simulink model "PMSM_FOC_Algorithm"  (R2024b)
settings: Solver=FixedStepAuto  StartTime=0.0  StopTime=1  FixedStep=1e-6  RelTol=1e-3
model workspace (MAT data in the model file):
  B = 0
  Current_Filter_On = 1
  F = 10000
  J = 5.8e-05
  Ls = 0.0005125
  Pn = 5
  Rs = 0.1445
  T_deadband = 3e-06
  Ts = 5e-05
  Vdc = 48
  id_ki = 0.01
  id_kp = 0.8
  iq_ki = 0.01
  iq_kp = 1.2
  psi_f = 0.0113
libraries: simulink x2, slpidlib x2, spsDCVoltageSourceLib x1, spsOnDelayLib x1, spsPermanentMagnetSynchronousMachineLib x1, spsTwoLevelConverterLib x1, spspowerguiLib x1
settings Model: Creator=A  LastModifiedBy=31904
settings OptimizationCC: ReuseModelBlockBuffer=off
settings ModelReferenceCC: EnableRefExpFcnMdlSchedulingChecks=on
settings RTWCC: GPUComputeCapability=3.5

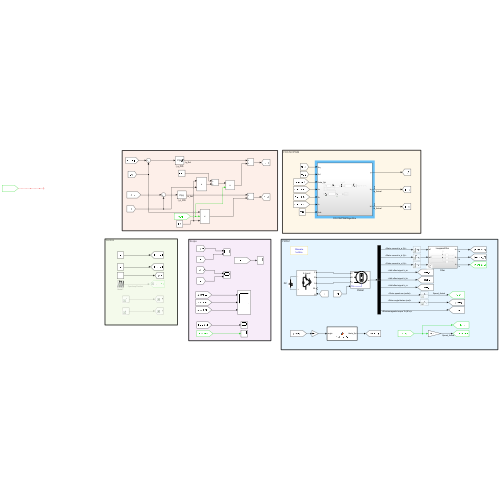
[thumbnail: Simulink's stored preview of the top-level diagram]
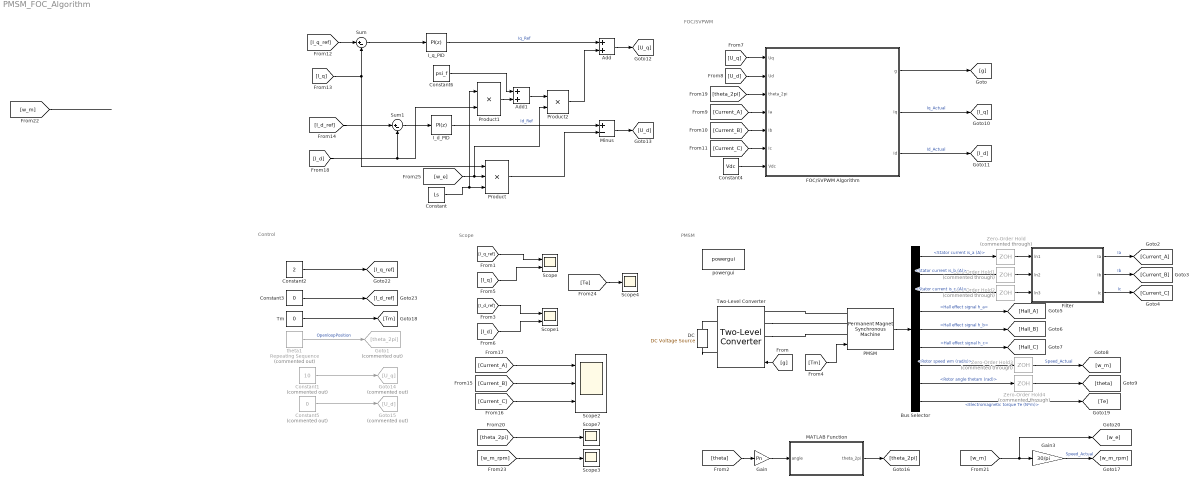
== system PMSM_FOC_Algorithm ==
  note: Scope
  note: Control
  note: FOC/SVPWM
  note: PMSM
  Add : Sum
  Add1 : Sum
  Bus Selector : BusSelector  OutputSignals=Stator current is_a (A),Stator current is_b (A),Stator current is_c (A),Hall effect signal h_a,Hall effect signal h_b,Hall effect signal h_c,Rotor speed wm (rad/s),Rotor angle thetam (rad),Electromagnetic torque Te (N*m)
  Constant : Constant  Value=Ls
  Constant1 : Constant  Commented=on  Value=10
  Constant2 : Constant  Value=2
  Constant3 : Constant  Value=0
  Constant4 : Constant  Value=Vdc
  Constant5 : Constant  Commented=on  Value=0
  Constant6 : Constant  Value=psi_f
  DC : spsDCVoltageSourceLib/DC Voltage Source  Amplitude=Vdc  Measurements=None
  FOC/SVPWM Algorithm : Subsystem
  Filter : Subsystem  Variant=on
  Gain : Gain  Gain=Pn
  Gain3 : Gain  Gain=30/pi
  Goto1 : Goto  Commented=on  GotoTag=theta_2pi
  Goto14 : Goto  Commented=on  GotoTag=U_q
  Goto15 : Goto  Commented=on  GotoTag=U_d
  I_d_PID : slpidlib/PID Controller  Controller=PI  Form=Parallel  TimeDomain=Discrete-time  UseExternalTs=off  SampleTime=-1  IntegratorMethod=Forward Euler  FilterMethod=Forward Euler  ControllerParametersSource=internal  P=id_kp  I=id_ki  UseKiTs=off  D=0  UseExternalDerivativeSource=off  N=100  UseFilter=on  TunerSelectOption=Transfer Function Based (PID Tuner App)  InitialConditionSource=internal  InitialConditionForIntegrator=0  InitialConditionForFilter=0  DifferentiatorICPrevScaledInput=0  ExternalReset=none  TrackingMode=off  Kt=1  LimitOutput=off  SatLimitsSource=internal  UpperSaturationLimit=10  LowerSaturationLimit=0  LinearizeAsGain=on  AntiWindupMode=none  Kb=1  LimitIntegrator=off  UpperIntegratorSaturationLimit=inf  LowerIntegratorSaturationLimit=-inf  POutMin=[]  POutMax=[]  IOutMin=[]  IOutMax=[]  DOutMin=[]  DOutMax=[]  NOutMin=[]  NOutMax=[]  SumOutMin=[]  SumOutMax=[]  SaturationOutMin=[]  SaturationOutMax=[]  PParamMin=[]  PParamMax=[]  IParamMin=[]  IParamMax=[]  DParamMin=[]  DParamMax=[]  NParamMin=[]  NParamMax=[]  KbParamMin=[]  KbParamMax=[]  KtParamMin=[]  KtParamMax=[]  KbOutMin=[]  KbOutMax=[]  KtOutMin=[]  KtOutMax=[]  IntegratorOutMin=[]  IntegratorOutMax=[]  FilterOutMin=[]  FilterOutMax=[]  SumI1OutMin=[]  SumI1OutMax=[]  SumI2OutMin=[]  SumI2OutMax=[]  SumI3OutMin=[]  SumI3OutMax=[]  SumI4OutMin=[]  SumI4OutMax=[]  SumDOutMin=[]  SumDOutMax=[]  DifferentiatorOutMin=[]  DifferentiatorOutMax=[]  FilterDiffOutCoefMin=[]  FilterDiffOutCoefMax=[]  ReciprocalOutMin=[]  ReciprocalOutMax=[]  SumDenOutMin=[]  SumDenOutMax=[]  SumNumOutMin=[]  SumNumOutMax=[]  DivideOutMin=[]  DivideOutMax=[]  UdiffTsProdOutMin=[]  UdiffTsProdOutMax=[]  NTsProdOutMin=[]  NTsProdOutMax=[]  UintegralTsProdOutMin=[]  UintegralTsProdOutMax=[]  UngainTsProdOutMin=[]  UngainTsProdOutMax=[]  ClampingZeroOutDataTypeStr=Inherit: Inherit via back propagation  ClampingZeroOutMin=[]  ClampingZeroOutMax=[]  FilterDenConstantOutDataTypeStr=Inherit: Inherit via back propagation  FilterDenConstantOutMin=[]  FilterDenConstantOutMax=[]  PCopyOutDataTypeStr=Inherit: Inherit via back propagation  PCopyOutMin=[]  PCopyOutMax=[]  NCopyOutDataTypeStr=Inherit: Inherit via back propagation  NCopyOutMin=[]  NCopyOutMax=[]  IntegratorContinuousStateAttributes=''  IntegratorStateMustResolveToSignalObject=off  IntegratorRTWStateStorageClass=Auto  FilterContinuousStateAttributes=''  FilterStateMustResolveToSignalObject=off  FilterRTWStateStorageClass=Auto  ParallelPVariant=InternalParameters  IdealPVariant=Disabled  IVariant=InternalParameters  DVariant=Disabled  IntegratorVariant=Discrete  SatVariant=Disabled  AWVariant=Passthrough  PCopyVariant=Disabled  TRVariant=Disabled  FdbkBlocksVariant=Forward  IdealPFdbkVariant=Disabled  SatFdbkVariant=Disabled  DerivativeFilterVariant=Disabled  NVariant=Disabled  NCopyVariant=Disabled_SignalSpec  FilterICVariant=Disabled  IntegratorICVariant=InternalICs  ExternalResetVariant=Disabled  TRSumVariant=Passthrough  SumFdbkVariant=Disabled  SumVariant=Sum_PI  TsampFilterVariant=InternalTs  TsampNgainVariant=Passthrough  TsampIntegralVariant=Disabled_SignalSpec  ExternalSaturationOutDataTypeStr=Inherit: Same as second input  DerivativeSourceVariant=Disabled  PreIntVariant=InternalPreInt
  I_q_PID : slpidlib/PID Controller  Controller=PI  Form=Parallel  TimeDomain=Discrete-time  UseExternalTs=off  SampleTime=-1  IntegratorMethod=Forward Euler  FilterMethod=Forward Euler  ControllerParametersSource=internal  P=iq_kp  I=iq_ki  UseKiTs=off  D=0  UseExternalDerivativeSource=off  N=100  UseFilter=on  TunerSelectOption=Transfer Function Based (PID Tuner App)  InitialConditionSource=internal  InitialConditionForIntegrator=0  InitialConditionForFilter=0  DifferentiatorICPrevScaledInput=0  ExternalReset=none  TrackingMode=off  Kt=1  LimitOutput=on  SatLimitsSource=internal  UpperSaturationLimit=Vdc  LowerSaturationLimit=0  LinearizeAsGain=on  AntiWindupMode=back-calculation  Kb=1  LimitIntegrator=off  UpperIntegratorSaturationLimit=inf  LowerIntegratorSaturationLimit=-inf  POutMin=[]  POutMax=[]  IOutMin=[]  IOutMax=[]  DOutMin=[]  DOutMax=[]  NOutMin=[]  NOutMax=[]  SumOutMin=[]  SumOutMax=[]  SaturationOutMin=[]  SaturationOutMax=[]  PParamMin=[]  PParamMax=[]  IParamMin=[]  IParamMax=[]  DParamMin=[]  DParamMax=[]  NParamMin=[]  NParamMax=[]  KbParamMin=[]  KbParamMax=[]  KtParamMin=[]  KtParamMax=[]  KbOutMin=[]  KbOutMax=[]  KtOutMin=[]  KtOutMax=[]  IntegratorOutMin=[]  IntegratorOutMax=[]  FilterOutMin=[]  FilterOutMax=[]  SumI1OutMin=[]  SumI1OutMax=[]  SumI2OutMin=[]  SumI2OutMax=[]  SumI3OutMin=[]  SumI3OutMax=[]  SumI4OutMin=[]  SumI4OutMax=[]  SumDOutMin=[]  SumDOutMax=[]  DifferentiatorOutMin=[]  DifferentiatorOutMax=[]  FilterDiffOutCoefMin=[]  FilterDiffOutCoefMax=[]  ReciprocalOutMin=[]  ReciprocalOutMax=[]  SumDenOutMin=[]  SumDenOutMax=[]  SumNumOutMin=[]  SumNumOutMax=[]  DivideOutMin=[]  DivideOutMax=[]  UdiffTsProdOutMin=[]  UdiffTsProdOutMax=[]  NTsProdOutMin=[]  NTsProdOutMax=[]  UintegralTsProdOutMin=[]  UintegralTsProdOutMax=[]  UngainTsProdOutMin=[]  UngainTsProdOutMax=[]  ClampingZeroOutDataTypeStr=Inherit: Inherit via back propagation  ClampingZeroOutMin=[]  ClampingZeroOutMax=[]  FilterDenConstantOutDataTypeStr=Inherit: Inherit via back propagation  FilterDenConstantOutMin=[]  FilterDenConstantOutMax=[]  PCopyOutDataTypeStr=Inherit: Inherit via back propagation  PCopyOutMin=[]  PCopyOutMax=[]  NCopyOutDataTypeStr=Inherit: Inherit via back propagation  NCopyOutMin=[]  NCopyOutMax=[]  IntegratorContinuousStateAttributes=''  IntegratorStateMustResolveToSignalObject=off  IntegratorRTWStateStorageClass=Auto  FilterContinuousStateAttributes=''  FilterStateMustResolveToSignalObject=off  FilterRTWStateStorageClass=Auto  ParallelPVariant=InternalParameters  IdealPVariant=Disabled  IVariant=InternalParameters  DVariant=Disabled  IntegratorVariant=Discrete  SatVariant=Enabled  AWVariant=BackCalculation  PCopyVariant=Disabled  TRVariant=Disabled  FdbkBlocksVariant=Forward  IdealPFdbkVariant=Disabled  SatFdbkVariant=Disabled  DerivativeFilterVariant=Disabled  NVariant=Disabled  NCopyVariant=Disabled_SignalSpec  FilterICVariant=Disabled  IntegratorICVariant=InternalICs  ExternalResetVariant=Disabled  TRSumVariant=Passthrough  SumFdbkVariant=Disabled  SumVariant=Sum_PI  TsampFilterVariant=InternalTs  TsampNgainVariant=Passthrough  TsampIntegralVariant=Disabled_SignalSpec  ExternalSaturationOutDataTypeStr=Inherit: Same as second input  DerivativeSourceVariant=Disabled  PreIntVariant=InternalPreInt
  MATLAB Function : MATLAB Function  TreatAsAtomicUnit=on
  Minus : Sum  Inputs=+-
  PMSM : spsPermanentMagnetSynchronousMachineLib/Permanent Magnet Synchronous Machine  NbPhases=3  FluxDistribution=Sinusoidal  RotorType=Round  MechanicalLoad=Torque Tm  PresetModel=No  ShowDetailedParameters=on  MeasurementBus=off  Resistance=Rs  Inductance=8.5e-3  dqInductances=[8.5e-3,8.5e-3]  La=Ls  MachineConstant=Flux linkage established by magnets (V.s)  Flux=psi_f  VoltageCst=10.248  TorqueCst=0.08475  Flat=120  Mechanical=[J B Pn 0]  PolePairs=4  InitialConditions=[0,0, 0,0]  InitialConditions5ph=[0 0 0 0 0 0]  RefAngle=Aligned with phase A axis (original Park)  IterativeDiscreteModel=Trapezoidal non iterative  TsBlock=-1  TsPowergui=0
  Product : Product  Inputs=3
  Product1 : Product
  Product2 : Product
  Scope : Scope  NumInputPorts=2
  Scope1 : Scope  NumInputPorts=2
  Scope2 : Scope  NumInputPorts=3
  Scope3 : Scope
  Scope4 : Scope
  Scope7 : Scope
  Sum : Sum  Inputs=|+-
  Sum1 : Sum  Inputs=|+-
  Tm : Constant  Value=0
  Two-Level Converter : spsTwoLevelConverterLib/Two-Level Converter  ModelType=Switching devices  Ron=1e-3  Rs=1e6  Cs=inf  Vforward=[0,0]  Ron_Diode=1e-3  Rs_Diode=1e6  Cs_Diode=inf  Vf_Diode=1e-3  Rs_CurrentSource=inf  Ron_ACsource=1e-3
  Zero-Order Hold{,1..4} (5 alike) : ZeroOrderHold  Commented=through  SampleTime=1/F
  powergui : spspowerguiLib/powergui  Priority=1  SimulationMode=Discrete  SampleTime=1e-6  frequency=60  Iterations=50  frequencyindice=0  Pbase=100e6  ErrMax=1e-4  UnitsV=kV  UnitsW=MW  buscounter=0  FunctionMessages=off  echomessages=off  EnableUseOfTLC=off  CurrentSourceSwitches=off  DisableSnubberDevices=off  DisableRonSwitches=off  DisableVfSwitches=off  DisplayEquations=off  AutomaticDiscreteSolvers=off  SolverType=Tustin/Backward Euler (TBE)  Interpol=off  ExternalGateDelay=off  methode=off  Ts=100  x0status=blocks  SPID=on  SwTol=0  HookPort=off  NonlinearTolerance=1e-4  nMaxIteration=100  ContinueOnMaxIteration=off  RestoreLinks=warning  ResistiveCurrentMeasurement=off  Frange=[0:2:500]  Ylog=off  Xlog=on  ShowGrid=off  save=off  variable=ZData  structure=0  ZoomFFT=off  StartTime=0.0  cycles=1  DisplayStyle=1  fundamental=60  FreqAxis=off  MaxFrequency=1000  frequencyindicesteady=1  RmsSteady=1  display=off
  theta1 : simulink/Sources/Repeating Sequence  Commented=on  rep_seq_t=[0 0.1]  rep_seq_y=[0 2*pi]
  wires:
  Constant4/1 -> FOC/SVPWM Algorithm/7(Vdc)
  [theta_2pi] -> FOC/SVPWM Algorithm/3(theta_2pi)
  FOC/SVPWM Algorithm/3(Id) -> [I_d]  "Id_Actual"
  [U_d] -> FOC/SVPWM Algorithm/2(Ud)
  [U_q] -> FOC/SVPWM Algorithm/1(Uq)
  [Current_A] -> FOC/SVPWM Algorithm/4(Ia)
  [Current_C] -> FOC/SVPWM Algorithm/6(Ic)
  FOC/SVPWM Algorithm/2(Iq) -> [I_q]  "Iq_Actual"
  [Current_B] -> FOC/SVPWM Algorithm/5(Ib)
  Zero-Order Hold4/1 -> [theta]
  Bus Selector/1 -> Zero-Order Hold/1  "<Stator current is_a (A)>"
  Zero-Order Hold/1 -> Filter/1(ln1)
  Zero-Order Hold1/1 -> Filter/2(ln2)
  Bus Selector/4 -> [Hall_A]  "<Hall effect signal h_a>"
  [theta] -> Gain/1
  Bus Selector/2 -> Zero-Order Hold1/1  "<Stator current is_b (A)>"
  [g] -> Two-Level Converter/1
  Bus Selector/3 -> Zero-Order Hold2/1  "<Stator current is_c (A)>"
  [Tm] -> PMSM/1
  Zero-Order Hold3/1 -> [w_m]  "Speed_Actual"
  Bus Selector/8 -> Zero-Order Hold4/1  "<Rotor angle thetam (rad)>"
  MATLAB Function/1(theta_2pi) -> [theta_2pi]
  Bus Selector/7 -> Zero-Order Hold3/1  "<Rotor speed wm (rad/s)>"
  PMSM/1 -> Bus Selector/1
  Bus Selector/5 -> [Hall_B]  "<Hall effect signal h_b>"
  Zero-Order Hold2/1 -> Filter/3(ln3)
  Bus Selector/6 -> [Hall_C]  "<Hall effect signal h_c>"
  Constant3/1 -> [I_d_ref]
  Constant2/1 -> [I_q_ref]
  [I_q_ref] -> Scope/1
  [I_q] -> Scope/2
  [I_d_ref] -> Scope1/1
  [I_d] -> Scope1/2
  I_q_PID/1 -> Add/1  "Iq_Ref"
  [I_q_ref] -> Sum/1
  [I_q] -> Sum/2, Product/1
  Sum/1 -> I_q_PID/1
  [Current_C] -> Scope2/3
  [Current_B] -> Scope2/2
  [Current_A] -> Scope2/1
  [theta_2pi] -> Scope7/1
  Filter/1(Ia) -> [Current_A]  "Ia"
  Filter/2(Ib) -> [Current_B]  "Ib"
  Filter/3(Ic) -> [Current_C]  "Ic"
  FOC/SVPWM Algorithm/1(g) -> [g]
  theta1/1 -> Goto1/1  "OpenloopPosition"
  Sum1/1 -> I_d_PID/1
  I_d_PID/1 -> Minus/1  "Id_Ref"
  [I_d] -> Product1/2, Sum1/2
  [I_d_ref] -> Sum1/1
  Constant5/1 -> Goto15/1
  Constant1/1 -> Goto14/1
  [w_m] -> [w_e], Gain3/1
  Gain3/1 -> [w_m_rpm]  "Speed_Actual"
  [w_m] -> ?
  [w_m_rpm] -> Scope3/1
  Gain/1 -> MATLAB Function/1(angle)
  Tm/1 -> [Tm]
  Bus Selector/9 -> [Te]  "<Electromagnetic torque Te (N*m)>"
  [Te] -> Scope4/1
  [w_e] -> Product2/2, Product/2
  Constant/1 -> Product1/1, Product/3
  Product/1 -> Minus/2
  Minus/1 -> [U_d]
  Product1/1 -> Add1/2
  Constant6/1 -> Add1/1
  Add1/1 -> Product2/1
  Product2/1 -> Add/2
  Add/1 -> [U_q]
  connections:
  DC/LConn1 -- Two-Level Converter/RConn2
  DC/RConn1 -- Two-Level Converter/RConn1
  PMSM/LConn3 -- Two-Level Converter/LConn3
  Two-Level Converter/LConn1 -- PMSM/LConn1
  Two-Level Converter/LConn2 -- PMSM/LConn2

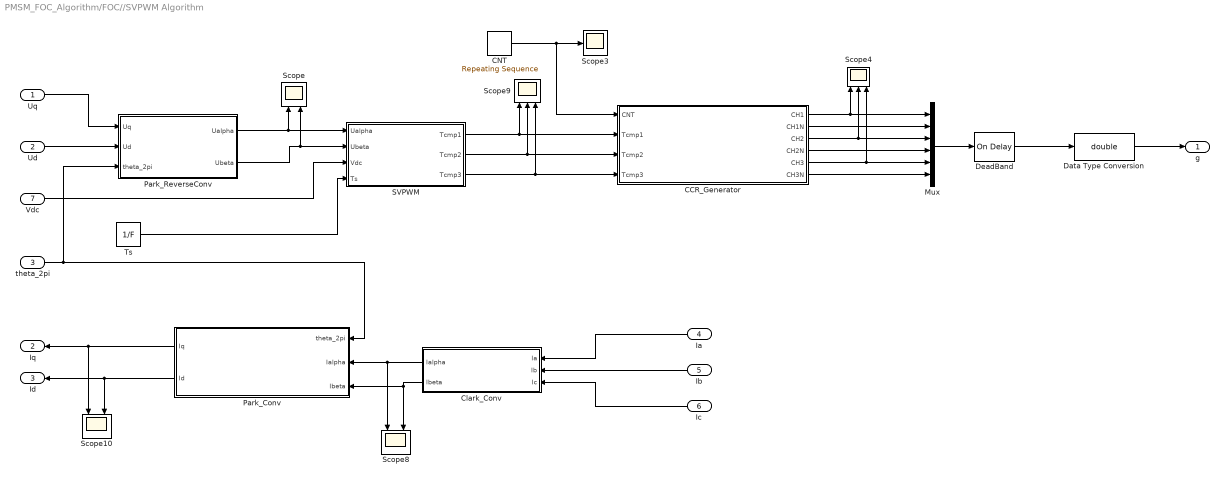
== system PMSM_FOC_Algorithm/FOC//SVPWM Algorithm ==
  Uq : Inport
  Ud : Inport  Port=2
  theta_2pi : Inport  Port=3
  Ia : Inport  Port=4
  Ib : Inport  Port=5
  Ic : Inport  Port=6
  Vdc : Inport  Port=7
  CCR_Generator : MATLAB Function  TreatAsAtomicUnit=on
  CNT : simulink/Sources/Repeating Sequence  rep_seq_t=[0 1/(2*F) 1/F]  rep_seq_y=[0 1/(2*F) 0]
  Clark_Conv : Subsystem
  Data Type Conversion : DataTypeConversion  OutDataTypeStr=double  SaturateOnIntegerOverflow=off  RndMeth=Floor
  DeadBand : spsOnDelayLib/On Delay  DelayType=On delay  delay=T_deadband  ic=0  Ts=0
  Mux : Mux  Inputs=6
  Park_Conv : Subsystem
  Park_ReverseConv : Subsystem
  SVPWM : Subsystem
  Scope : Scope  NumInputPorts=2
  Scope10 : Scope  NumInputPorts=2
  Scope3 : Scope
  Scope4 : Scope  NumInputPorts=3
  Scope8 : Scope  NumInputPorts=2
  Scope9 : Scope  NumInputPorts=3
  Ts : Constant  Value=1/F
  g : Outport
  Iq : Outport  Port=2
  Id : Outport  Port=3
  wires:
  Uq/1 -> Park_ReverseConv/1(Uq)
  SVPWM/3(Tcmp3) -> CCR_Generator/4(Tcmp3), Scope9/3
  Clark_Conv/1(Ialpha) -> Park_Conv/2(Ialpha), Scope8/1
  CCR_Generator/3(CH2) -> Mux/3, Scope4/2
  SVPWM/2(Tcmp2) -> CCR_Generator/3(Tcmp2), Scope9/2
  CCR_Generator/2(CH1N) -> Mux/2
  theta_2pi/1 -> Park_Conv/1(theta_2pi), Park_ReverseConv/3(theta_2pi)
  CCR_Generator/5(CH3) -> Mux/5, Scope4/3
  SVPWM/1(Tcmp1) -> CCR_Generator/2(Tcmp1), Scope9/1
  Clark_Conv/2(Ibeta) -> Park_Conv/3(Ibeta), Scope8/2
  CCR_Generator/4(CH2N) -> Mux/4
  Park_ReverseConv/1(Ualpha) -> SVPWM/1(Ualpha), Scope/1
  CCR_Generator/6(CH3N) -> Mux/6
  Mux/1 -> DeadBand/1
  Park_ReverseConv/2(Ubeta) -> Scope/2, SVPWM/2(Ubeta)
  CNT/1 -> Scope3/1, CCR_Generator/1(CNT)
  Park_Conv/2(Id) -> Scope10/2, Id/1
  CCR_Generator/1(CH1) -> Mux/1, Scope4/1
  Ud/1 -> Park_ReverseConv/2(Ud)
  Park_Conv/1(Iq) -> Scope10/1, Iq/1
  Data Type Conversion/1 -> g/1
  Vdc/1 -> SVPWM/3(Vdc)
  Ic/1 -> Clark_Conv/3(Ic)
  Ib/1 -> Clark_Conv/2(Ib)
  Ia/1 -> Clark_Conv/1(Ia)
  Ts/1 -> SVPWM/4(Ts)
  DeadBand/1 -> Data Type Conversion/1

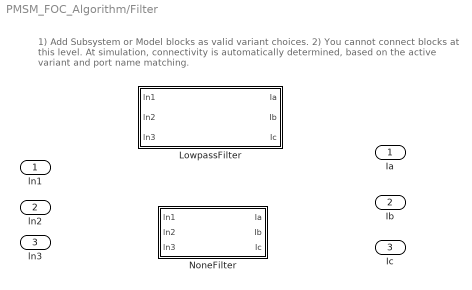
== system PMSM_FOC_Algorithm/Filter ==
  note: 1) Add Subsystem or Model blocks as valid variant choices.
      | 2) You cannot connect blocks at this level. At simulation, connectivity is automatically
      | determined, based on the active variant and port name matching.
  ln1 : Inport
  ln2 : Inport  Port=2
  ln3 : Inport  Port=3
  LowpassFilter : Subsystem  VariantControl=Current_Filter_On==1
  NoneFilter : Subsystem  VariantControl=Current_Filter_On==0
  Ia : Outport
  Ib : Outport  Port=2
  Ic : Outport  Port=3

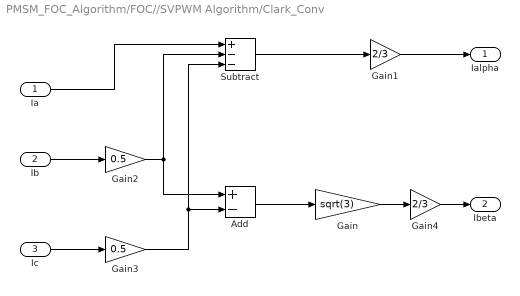
== system PMSM_FOC_Algorithm/FOC//SVPWM Algorithm/Clark_Conv ==
  Ia : Inport
  Ib : Inport  Port=2
  Ic : Inport  Port=3
  Add : Sum  Inputs=+-  OutDataTypeStr=double
  Gain : Gain  Gain=sqrt(3)  ParamDataTypeStr=double
  Gain1 : Gain  Gain=2/3
  Gain2 : Gain  Gain=0.5
  Gain3 : Gain  Gain=0.5
  Gain4 : Gain  Gain=2/3
  Subtract : Sum  Inputs=+--  OutDataTypeStr=double
  Ialpha : Outport
  Ibeta : Outport  Port=2
  wires:
  Ia/1 -> Subtract/1
  Ib/1 -> Gain2/1
  Add/1 -> Gain/1
  Gain/1 -> Gain4/1
  Ic/1 -> Gain3/1
  Gain2/1 -> Subtract/2, Add/1
  Gain3/1 -> Subtract/3, Add/2
  Subtract/1 -> Gain1/1
  Gain1/1 -> Ialpha/1
  Gain4/1 -> Ibeta/1

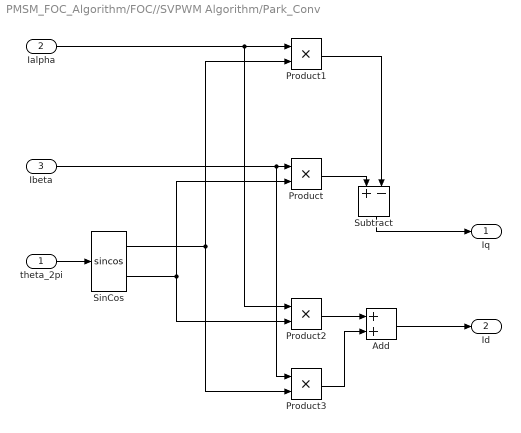
== system PMSM_FOC_Algorithm/FOC//SVPWM Algorithm/Park_Conv ==
  theta_2pi : Inport
  Ialpha : Inport  Port=2
  Ibeta : Inport  Port=3
  Add : Sum
  Product{,1..3} (4 alike) : Product
  SinCos : Trigonometry  Operator=sincos
  Subtract : Sum  Inputs=+-
  Iq : Outport
  Id : Outport  Port=2
  wires:
  Ialpha/1 -> Product1/1, Product2/1
  Ibeta/1 -> Product3/1, Product/1
  theta_2pi/1 -> SinCos/1
  SinCos/2 -> Product2/2, Product/2
  SinCos/1 -> Product3/2, Product1/2
  Product1/1 -> Subtract/2
  Subtract/1 -> Iq/1
  Product/1 -> Subtract/1
  Product2/1 -> Add/1
  Product3/1 -> Add/2
  Add/1 -> Id/1

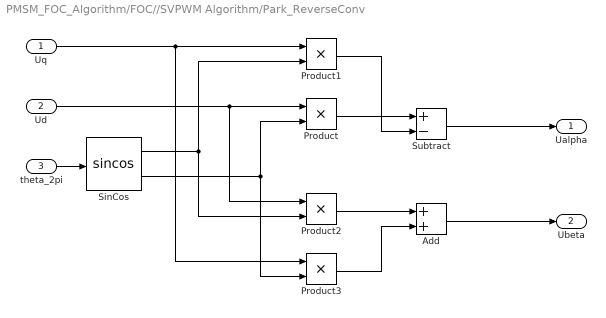
== system PMSM_FOC_Algorithm/FOC//SVPWM Algorithm/Park_ReverseConv ==
  Uq : Inport
  Ud : Inport  Port=2
  theta_2pi : Inport  Port=3
  Add : Sum
  Product{,1..3} (4 alike) : Product
  SinCos : Trigonometry  Operator=sincos
  Subtract : Sum  Inputs=+-
  Ualpha : Outport
  Ubeta : Outport  Port=2
  wires:
  Uq/1 -> Product3/1, Product1/1
  Ud/1 -> Product2/1, Product/1
  SinCos/2 -> Product3/2, Product/2
  Product/1 -> Subtract/1
  SinCos/1 -> Product2/2, Product1/2
  Product1/1 -> Subtract/2
  Subtract/1 -> Ualpha/1
  Product2/1 -> Add/1
  Product3/1 -> Add/2
  Add/1 -> Ubeta/1
  theta_2pi/1 -> SinCos/1

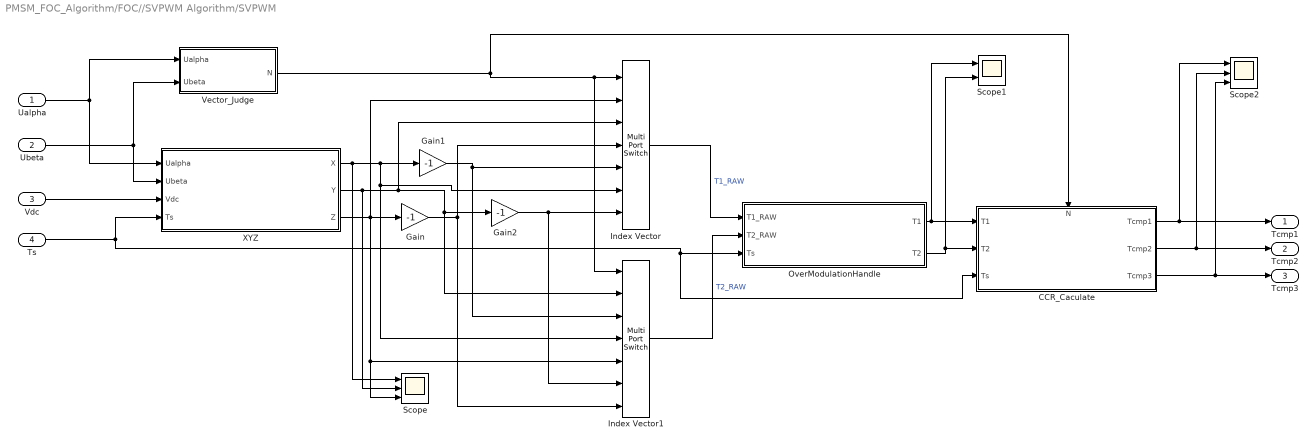
== system PMSM_FOC_Algorithm/FOC//SVPWM Algorithm/SVPWM ==
  Ualpha : Inport
  Ubeta : Inport  Port=2
  Vdc : Inport  Port=3
  Ts : Inport  Port=4
  CCR_Caculate : Subsystem
      settings: PortSchema="{\"entries\":[{\"content\":{\"sides\":[{\"content\":{\"connectorIds\":[\"In1\",\"In2\",\"In3\"]},\"type\":\"ConnectorPlacement.EquallySpacedRectSide\",\"uuid\":\"41d89106-695f-4d7e-9c99-c52170b99868\"},{\"content\":{\"connectorIds\":[\"Out1\",\"Out2\",\"Out3\"],\"side\":\"RIGHT\"},\"type\":\"ConnectorPlacement.EquallySpacedRectSide\",\"uuid\":\"0fa1e6b9-7088-4c16-9dd3-c016449aae3e\"},{\"content\":{\"connectorIds\":[\"In4\"],\"side\":\"TOP\"},\"type\":\"ConnectorPlacement.EquallySpacedRectSide\",\"uuid\":\"6b702c00-29ab-49c7-a344-eb6fce3368af\"}]},\"type\":\"ConnectorPlacement.EquallySpacedConnector\",\"uuid\":\"c2f99839-550c-47c5-98fa-a115626cfb71\"}],\"packageUris\":[\"http://schema.mathworks.com/mf0/Connector/R2020b\"],\"version\":\"1.0\"}"
  Gain : Gain  Gain=-1
  Gain1 : Gain  Gain=-1
  Gain2 : Gain  Gain=-1
  Index Vector : MultiPortSwitch  Inputs=6  SaturateOnIntegerOverflow=off  InputSameDT=off
  Index Vector1 : MultiPortSwitch  Inputs=6  SaturateOnIntegerOverflow=off  InputSameDT=off
  OverModulationHandle : MATLAB Function  TreatAsAtomicUnit=on
  Scope : Scope  NumInputPorts=3
  Scope1 : Scope  NumInputPorts=2
  Scope2 : Scope  NumInputPorts=3
  Vector_Judge : Subsystem
  XYZ : Subsystem
  Tcmp1 : Outport
  Tcmp2 : Outport  Port=2
  Tcmp3 : Outport  Port=3
  wires:
  Ualpha/1 -> Vector_Judge/1(Ualpha), XYZ/1(Ualpha)
  Ubeta/1 -> Vector_Judge/2(Ubeta), XYZ/2(Ubeta)
  Vdc/1 -> XYZ/3(Vdc)
  Ts/1 -> CCR_Caculate/3(Ts), OverModulationHandle/3(Ts), XYZ/4(Ts)
  Vector_Judge/1(N) -> Index Vector1/1, Index Vector/1, CCR_Caculate/4(N)
  Index Vector1/1 -> OverModulationHandle/2(T2_RAW)  "T2_RAW"
  XYZ/3(Z) -> Scope/3, Index Vector1/5, Index Vector/2, Gain/1
  XYZ/2(Y) -> Scope/2, Index Vector1/2, Gain2/1, Index Vector/3
  Gain/1 -> Index Vector1/7, Index Vector/4
  XYZ/1(X) -> Scope/1, Index Vector1/4, Index Vector/6, Gain1/1
  Gain1/1 -> Index Vector1/3, Index Vector/5
  Gain2/1 -> Index Vector1/6, Index Vector/7
  Index Vector/1 -> OverModulationHandle/1(T1_RAW)  "T1_RAW"
  OverModulationHandle/1(T1) -> CCR_Caculate/1(T1), Scope1/1
  OverModulationHandle/2(T2) -> Scope1/2, CCR_Caculate/2(T2)
  CCR_Caculate/1(Tcmp1) -> Tcmp1/1, Scope2/1
  CCR_Caculate/2(Tcmp2) -> Tcmp2/1, Scope2/2
  CCR_Caculate/3(Tcmp3) -> Tcmp3/1, Scope2/3

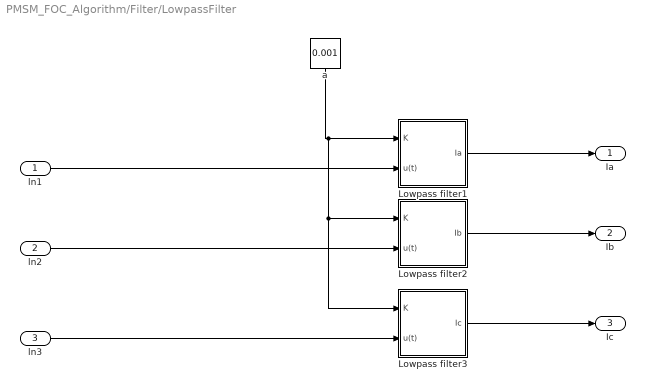
== system PMSM_FOC_Algorithm/Filter/LowpassFilter ==
  ln1 : Inport
  ln2 : Inport  Port=2
  ln3 : Inport  Port=3
  Lowpass filter1 : Subsystem
  Lowpass filter2 : Subsystem
  Lowpass filter3 : Subsystem
  a : Constant  Value=0.001
  Ia : Outport
  Ib : Outport  Port=2
  Ic : Outport  Port=3
  wires:
  ln2/1 -> Lowpass filter2/2(u(t))
  a/1 -> Lowpass filter3/1(K), Lowpass filter2/1(K), Lowpass filter1/1(K)
  ln1/1 -> Lowpass filter1/2(u(t))
  Lowpass filter1/1(Ia) -> Ia/1
  Lowpass filter2/1(Ib) -> Ib/1
  Lowpass filter3/1(Ic) -> Ic/1
  ln3/1 -> Lowpass filter3/2(u(t))

== system PMSM_FOC_Algorithm/Filter/NoneFilter ==
  ln1 : Inport
  ln2 : Inport  Port=2
  ln3 : Inport  Port=3
  Ia : Outport
  Ib : Outport  Port=2
  Ic : Outport  Port=3
  wires:
  ln1/1 -> Ia/1
  ln2/1 -> Ib/1
  ln3/1 -> Ic/1

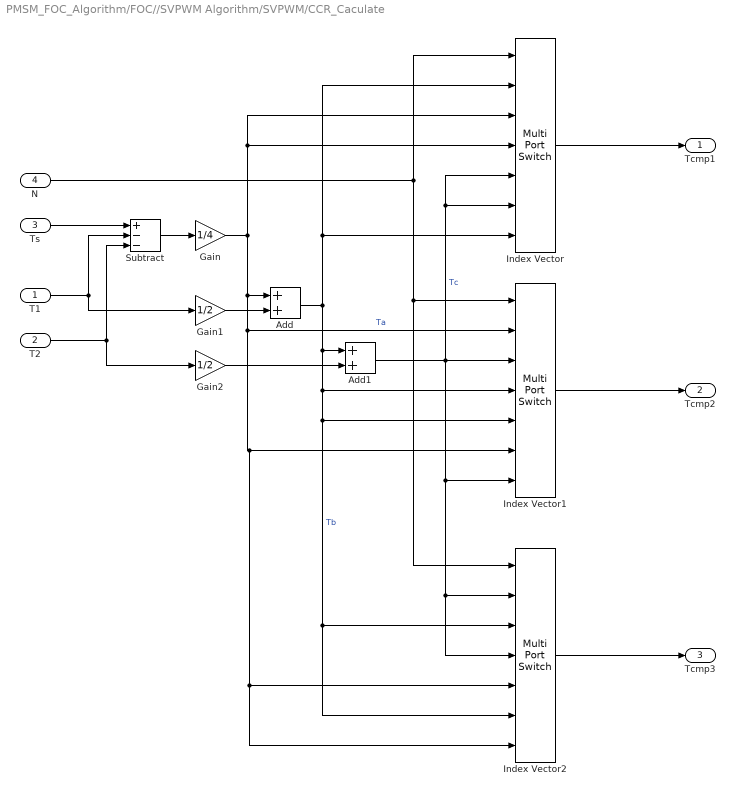
== system PMSM_FOC_Algorithm/FOC//SVPWM Algorithm/SVPWM/CCR_Caculate ==
  T1 : Inport
  T2 : Inport  Port=2
  Ts : Inport  Port=3
  N : Inport  Port=4
  Add : Sum
  Add1 : Sum
  Gain : Gain  Gain=1/4
  Gain1 : Gain  Gain=1/2
  Gain2 : Gain  Gain=1/2
  Index Vector : MultiPortSwitch  Inputs=6  SaturateOnIntegerOverflow=off  InputSameDT=off
  Index Vector1 : MultiPortSwitch  Inputs=6  SaturateOnIntegerOverflow=off  InputSameDT=off
  Index Vector2 : MultiPortSwitch  Inputs=6  SaturateOnIntegerOverflow=off  InputSameDT=off
  Subtract : Sum  Inputs=+--
  Tcmp1 : Outport
  Tcmp2 : Outport  Port=2
  Tcmp3 : Outport  Port=3
  wires:
  Ts/1 -> Subtract/1
  T1/1 -> Gain1/1, Subtract/2
  T2/1 -> Gain2/1, Subtract/3
  Subtract/1 -> Gain/1
  Gain/1 -> Index Vector2/7, Index Vector2/5, Index Vector1/6, Index Vector1/2, Add/1, Index Vector/4, Index Vector/3  "Ta"
  Gain1/1 -> Add/2
  Add/1 -> Index Vector1/5, Index Vector2/6, Index Vector2/3, Index Vector1/4, Add1/1, Index Vector/7, Index Vector/2  "Tb"
  Gain2/1 -> Add1/2
  Add1/1 -> Index Vector2/4, Index Vector2/2, Index Vector1/7, Index Vector1/3, Index Vector/6, Index Vector/5  "Tc"
  N/1 -> Index Vector2/1, Index Vector1/1, Index Vector/1
  Index Vector/1 -> Tcmp1/1
  Index Vector1/1 -> Tcmp2/1
  Index Vector2/1 -> Tcmp3/1

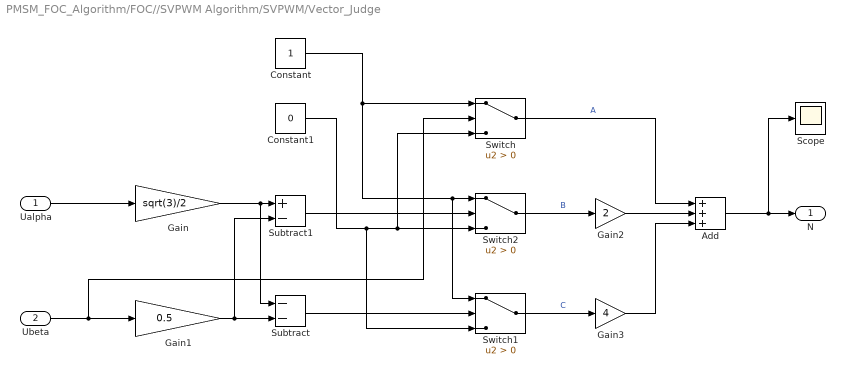
== system PMSM_FOC_Algorithm/FOC//SVPWM Algorithm/SVPWM/Vector_Judge ==
  Ualpha : Inport
  Ubeta : Inport  Port=2
  Add : Sum  Inputs=+++
  Constant : Constant
  Constant1 : Constant  Value=0
  Gain : Gain  Gain=sqrt(3)/2
  Gain1 : Gain  Gain=0.5
  Gain2 : Gain  Gain=2
  Gain3 : Gain  Gain=4
  Scope : Scope
  Subtract : Sum  Inputs=--
  Subtract1 : Sum  Inputs=+-
  Switch : Switch  Criteria=u2 > Threshold  SaturateOnIntegerOverflow=off  InputSameDT=off
  Switch1 : Switch  Criteria=u2 > Threshold  SaturateOnIntegerOverflow=off  InputSameDT=off
  Switch2 : Switch  Criteria=u2 > Threshold  SaturateOnIntegerOverflow=off  InputSameDT=off
  N : Outport
  wires:
  Ualpha/1 -> Gain/1
  Ubeta/1 -> Gain1/1, Switch/2
  Switch/1 -> Add/1  "A"
  Switch1/1 -> Gain3/1  "C"
  Constant1/1 -> Switch2/3, Switch/3, Switch1/3
  Constant/1 -> Switch2/1, Switch1/1, Switch/1
  Switch2/1 -> Gain2/1  "B"
  Gain3/1 -> Add/3
  Add/1 -> Scope/1, N/1
  Gain2/1 -> Add/2
  Gain/1 -> Subtract/1, Subtract1/1
  Gain1/1 -> Subtract/2, Subtract1/2
  Subtract1/1 -> Switch2/2
  Subtract/1 -> Switch1/2

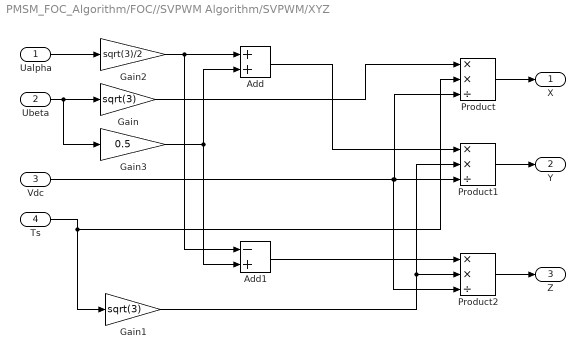
== system PMSM_FOC_Algorithm/FOC//SVPWM Algorithm/SVPWM/XYZ ==
  Ualpha : Inport
  Ubeta : Inport  Port=2
  Vdc : Inport  Port=3
  Ts : Inport  Port=4
  Add : Sum
  Add1 : Sum  Inputs=-+
  Gain : Gain  Gain=sqrt(3)
  Gain1 : Gain  Gain=sqrt(3)
  Gain2 : Gain  Gain=sqrt(3)/2
  Gain3 : Gain  Gain=0.5
  Product : Product  Inputs=**/
  Product1 : Product  Inputs=**/
  Product2 : Product  Inputs=**/
  X : Outport
  Y : Outport  Port=2
  Z : Outport  Port=3
  wires:
  Ualpha/1 -> Gain2/1
  Gain/1 -> Product/1
  Ubeta/1 -> Gain3/1, Gain/1
  Ts/1 -> Product/2, Gain1/1
  Vdc/1 -> Product1/3, Product/3, Product2/3
  Product/1 -> X/1
  Gain2/1 -> Add1/1, Add/1
  Gain3/1 -> Add/2, Add1/2
  Add/1 -> Product1/1
  Gain1/1 -> Product2/2, Product1/2
  Product1/1 -> Y/1
  Add1/1 -> Product2/1
  Product2/1 -> Z/1

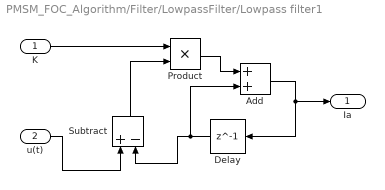
== system PMSM_FOC_Algorithm/Filter/LowpassFilter/Lowpass filter1 ==
  K : Inport
  u(t) : Inport  Port=2
  Add : Sum
  Delay : Delay  DelayLength=1
  Product : Product
  Subtract : Sum  Inputs=+-
  Ia : Outport
  wires:
  Add/1 -> Ia/1, Delay/1
  Product/1 -> Add/1
  Subtract/1 -> Product/2
  Delay/1 -> Subtract/2, Add/2
  K/1 -> Product/1
  u(t)/1 -> Subtract/1

== system PMSM_FOC_Algorithm/Filter/LowpassFilter/Lowpass filter2 ==
  K : Inport
  u(t) : Inport  Port=2
  Add : Sum
  Delay : Delay  DelayLength=1
  Product : Product
  Subtract : Sum  Inputs=+-
  Ib : Outport
  wires:
  u(t)/1 -> Subtract/1
  K/1 -> Product/1
  Delay/1 -> Add/2, Subtract/2
  Subtract/1 -> Product/2
  Product/1 -> Add/1
  Add/1 -> Delay/1, Ib/1

== system PMSM_FOC_Algorithm/Filter/LowpassFilter/Lowpass filter3 ==
  K : Inport
  u(t) : Inport  Port=2
  Add : Sum
  Delay : Delay  DelayLength=1
  Product : Product
  Subtract : Sum  Inputs=+-
  Ic : Outport
  wires:
  Add/1 -> Ic/1, Delay/1
  Product/1 -> Add/1
  Subtract/1 -> Product/2
  Delay/1 -> Subtract/2, Add/2
  K/1 -> Product/1
  u(t)/1 -> Subtract/1

== matlab function PMSM_FOC_Algorithm/MATLAB Function ==
  data: angle input; theta_2pi output
function theta_2pi = Angle_Conv(angle)

theta_2pi=mod(angle,2*pi);

== matlab function PMSM_FOC_Algorithm/FOC//SVPWM Algorithm/CCR_Generator ==
  data: CNT input; Tcmp1 input; Tcmp2 input; Tcmp3 input; CH1 output; CH1N output; CH2 output; CH2N output; CH3 output; CH3N output
function[CH1,CH1N,CH2,CH2N,CH3,CH3N] = CCR_Generator(CNT,Tcmp1, Tcmp2, Tcmp3)

if (CNT<Tcmp1)
    CH1=0;
    CH1N=1;
else
    CH1=1;
    CH1N=0;
end
if (CNT<Tcmp2)
    CH2=0;
    CH2N=1;
else
    CH2=1;
    CH2N=0;
end
if (CNT<Tcmp3)
    CH3=0;
    CH3N=1;
else
    CH3=1;
    CH3N=0;
end
end

== matlab function PMSM_FOC_Algorithm/FOC//SVPWM Algorithm/SVPWM/OverModulationHandle ==
  data: T1_RAW input; T2_RAW input; T1 output; T2 output; Ts input
function [T1,T2] = OverModulationHandle(T1_RAW, T2_RAW, Ts)
if((T1_RAW+T2_RAW)>Ts)
    T1=T1_RAW/(T1_RAW+T2_RAW)*Ts;
    T2=T2_RAW/(T1_RAW+T2_RAW)*Ts;
else
    T1=T1_RAW;
    T2=T2_RAW;
end
end
